simulink model "simulink_drone_offline_kalman"  (R2024b)
settings: Solver=VariableStepAuto  StartTime=0.0  StopTime=20  RelTol=1e-3
values from neighbouring files (symbols this model uses):
  A = A_numeric    [calculate_kalman_gain.m]    (also in expanded_drone_dynamics.m = [1 0 0 0 0 0 dt 0 0 0 0 0 0.5*(dt^2) 0 0 0 0 0; lqr_computation.m = jacobian(f, X); new_strategy.m = jacobian(f, X); new_strategy_integrated.m = jacobian(f, X))
  B = B_numeric    [calculate_kalman_gain.m]    (also in lqr_computation.m = jacobian(f, U); new_strategy.m = jacobian(f, U); new_strategy_integrated.m = jacobian(f, U); offline_kalman_expanded.m)
  barometer_sample_time = 1/100    (= 0.01)    [simulink_vars.m]
  barometer_variance = [0.0625]    [simulink_vars.m]
  C = C_imu    [offline_kalman_expanded.m]
  C_barometer = [0 0 1 0 0 0 0 0 0 0 0 0 0 0 0 0 0 0]    [offline_kalman_expanded.m]
  C_gps = [1 0 0 0 0 0 0 0 0 0 0 0 0 0 0 0 0 0 ... (first row only)    [offline_kalman_expanded.m]
  g = params.g    [drone_dynamics.m]    (also in expanded_drone_dynamics.m; lqr_computation.m = 9.807; new_strategy.m; new_strategy_integrated.m)
  G_hov = [ 0 0 0 0 0 0 1 0 ]    [lqr_computation.m]    (also in new_strategy.m = [1 0 0 0 0 0 0 0]; new_strategy_integrated.m = [1 0 0 0 0 0 0 0])
  G_pos = [ 1 0 0 0 ... (first row only)    [lqr_computation.m]    (also in new_strategy.m = [1 0 0 0; new_strategy_integrated.m = [1 0 0 0)
  gps_sample_time = 1/20    (= 0.05)    [simulink_vars.m]
  gps_variance = 0.0025 * ones(1,3)    [simulink_vars.m]
  imu_drift = [0.0,0.0,0.0,0.00,0.00,0.00,0.0,0.0,0.0]    [simulink_vars.m]
  imu_sample_time = 1/100    (= 0.01)    [simulink_vars.m]
  imu_variance = [0.0037,0.0037,0.0037,0.1225,0.1225,0.1225,0.0029,0.0029,0.0029]    [simulink_vars.m]
  K_att = lqr(sys_red_int, Q, R)    [new_strategy.m]    (also in new_strategy_integrated.m)
  K_hor = lqr(sys_hor_int, Q_hor, R_hor)    [new_strategy.m]    (also in new_strategy_integrated.m)
  kf = round( kf, 5 )    [offline_kalman_expanded.m]
  kf_100 = round(kf_100, 5)    [calculate_kalman_gain.m]    (also in offline_kalman_expanded.m = round( kf_100, 5 ))
  kf_20 = round(kf_20, 5)    [calculate_kalman_gain.m]    (also in offline_kalman_expanded.m = round( kf_20, 5 ))
  params = struct()    [simulink_vars.m]
  params_control = [m; Jx; Jy; Jz; c; r; g]    [new_strategy.m]    (also in new_strategy_integrated.m)
  stationary_wt = sqrt(weight/(Kt * 2))    [simulink_vars.m]
  X0 = [0;0;0; 0;0;0; 0;0;0; 0;0;0]    [new_strategy.m]    (also in new_strategy_integrated.m; simulink_vars.m = [0;0;3; 0;0;0; 0;0;0; 0;0;0])
undefined symbols (not defined in the file or in its folder): B_kinematic
settings Model: Creator=dp271  LastModifiedBy=dp271

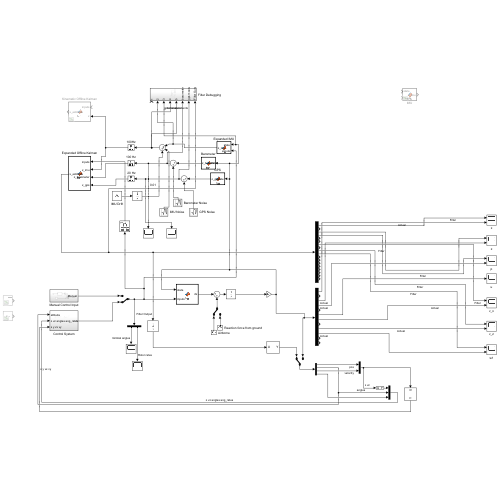
[thumbnail: Simulink's stored preview of the top-level diagram]
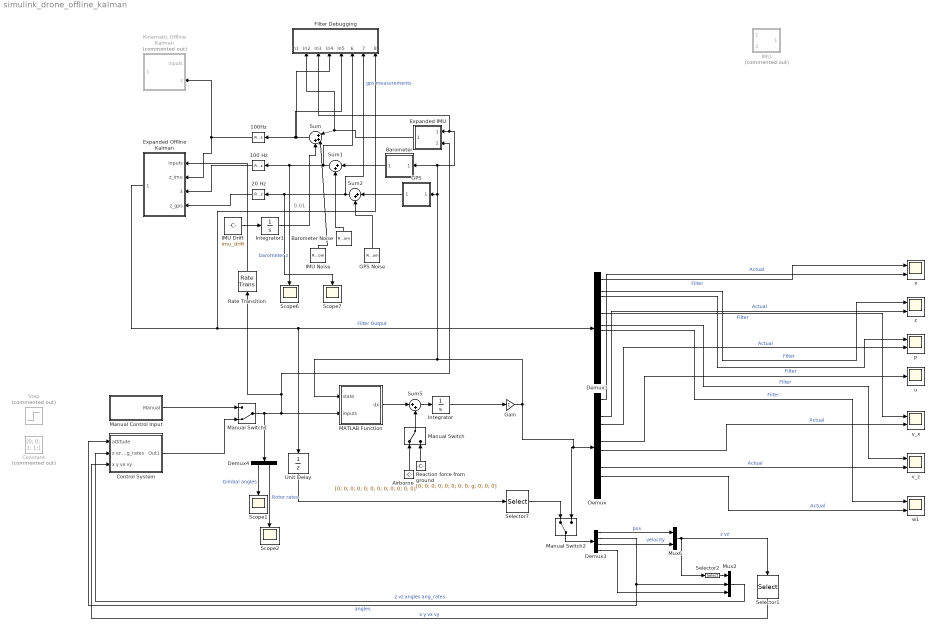
== system simulink_drone_offline_kalman ==
  note: 0.01
  " 20 Hz" : RateTransition  OutPortSampleTime=gps_sample_time
  100 Hz : RateTransition  OutPortSampleTime=barometer_sample_time
  100Hz : RateTransition  OutPortSampleTime=imu_sample_time
  Airborne : Constant  Value=[0; 0; 0; 0; 0; 0; 0; 0; 0; 0; 0; 0]
  Barometer : MATLAB Function  TreatAsAtomicUnit=on
  Barometer Noise : RandomNumber  Variance=barometer_variance  SampleTime=barometer_sample_time
  Constant : Constant  Commented=on  Value=[0; 0; 1; 1;]
  Control System : Subsystem
  Demux : Demux  Outputs=12
  Demux1 : Demux  Outputs=18
  Demux3 : Demux
  Demux4 : Demux  Outputs=2
  Expanded IMU : MATLAB Function  TreatAsAtomicUnit=on
  Expanded Offline Kalman : MATLAB Function  TreatAsAtomicUnit=on
  Filter Debugging : Subsystem
  GPS : MATLAB Function  TreatAsAtomicUnit=on
  GPS Noise : RandomNumber  Mean=zeros(3,1)  Variance=gps_variance  SampleTime=gps_sample_time
  Gain : Gain
  IMU : MATLAB Function  Commented=on  TreatAsAtomicUnit=on
  IMU Drift : Constant  Value=imu_drift  SampleTime=imu_sample_time
  IMU Noise : RandomNumber  Mean=zeros(9,1)  Variance=imu_variance  SampleTime=imu_sample_time
  Integrator : Integrator  InitialCondition=zeros(12,1)
  Integrator1 : Integrator  InitialCondition=zeros(9,1)
  Kinematic Offline Kalman : MATLAB Function  Commented=on  TreatAsAtomicUnit=on
  MATLAB Function : MATLAB Function  TreatAsAtomicUnit=on
  Manual Control Input : Subsystem
  Manual Switch : ManualSwitch
  Manual Switch1 : ManualSwitch  CurrentSetting=0
  Manual Switch2 : ManualSwitch
  Mux2 : Mux  Inputs=3
  Mux6 : Mux  Inputs=2
  Rate Transition : RateTransition  OutPortSampleTime=0.01
  Reaction force from ground : Constant  Value=[0; 0; 0; 0; 0; 0; 0; 0; g; 0; 0; 0]
  Scope{1..2,6..7} (4 alike) : Scope
  Selector1 : Selector  InputPortWidth=6  IndexOptions=Index vector (dialog)  Indices=[1 2 4 5]  OutputSizes=1
  Selector2 : Selector  InputPortWidth=6  IndexOptions=Index vector (dialog)  Indices=[3 6]  OutputSizes=1
  Selector7 : Selector  InputPortWidth=18  IndexOptions=Index vector (dialog)  Indices=[1 2 3 4 5 6 7 8 9 10 11 12]  OutputSizes=1
  Step : Step  Commented=on  Time=5  Before=stationary_wt  After=stationary_wt  SampleTime=0
  Sum : Sum  Inputs=|+++
  Sum1 : Sum  Inputs=|++
  Sum2 : Sum  Inputs=|++
  Sum5 : Sum  Inputs=|++
  Unit Delay : UnitDelay  InitialCondition=zeros(18,1)  SampleTime=0.01  HasFrameUpgradeWarning=on
  p : Scope  NumInputPorts=2
  u : Scope
  v_x : Scope  NumInputPorts=2
  v_z : Scope  NumInputPorts=2
  w1 : Scope  NumInputPorts=2
  x : Scope  NumInputPorts=2
  z : Scope  NumInputPorts=2
  wires:
  " 20 Hz"/1 -> Expanded Offline Kalman/4(z_gps)
  Demux1/1 -> x/1  "Filter"
  Demux/3 -> z/2  "Actual"
  Demux1/7 -> v_x/1  "Filter"
  Demux1/3 -> z/1  "Filter"
  IMU Drift/1 -> Integrator1/1
  Sum1/1 -> 100 Hz/1, Scope6/1, Filter Debugging/6(barometer z)  "barometer z"
  Demux/4 -> p/2  "Actual"
  Demux1/9 -> v_z/1  "Filter"
  Integrator1/1 -> Sum/3
  Barometer Noise/1 -> Sum1/2
  Demux/7 -> v_x/2  "Actual"
  Sum2/1 -> Filter Debugging/7(gps measurements), Scope7/1, " 20 Hz"/1  "gps measurements"
  GPS Noise/1 -> Sum2/2
  Demux/1 -> x/2  "Actual"
  Demux/9 -> v_z/2  "Actual"
  Sum/1 -> 100Hz/1, Filter Debugging/5(In5), Filter Debugging/4(In4)
  Demux1/4 -> p/1  "Filter"
  IMU Noise/1 -> Sum/2
  GPS/1(z_gps) -> Sum2/1
  100Hz/1 -> Expanded Offline Kalman/2(z_imu), Kinematic Offline Kalman/2(z)
  Expanded Offline Kalman/1(x_estimate) -> Demux1/1, Unit Delay/1, Filter Debugging/8(Filter Output)  "Filter Output"
  Barometer/1(z_barometer) -> Sum1/1
  100 Hz/1 -> Expanded Offline Kalman/3(z_barometer)
  Rate Transition/1 -> Expanded Offline Kalman/1(inputs)
  Gain/1 -> Demux/1, Manual Switch2/2, GPS/1(state), Filter Debugging/3(In3), Expanded IMU/1(state), Barometer/1(state), MATLAB Function/1(state)
  Demux1/10 -> w1/1  "Filter"
  Demux/10 -> w1/2  "Actual"
  MATLAB Function/1(dx) -> Sum5/1
  Sum5/1 -> Integrator/1
  Expanded IMU/1(z_imu) -> Filter Debugging/2(In2), Sum/1
  Integrator/1 -> Gain/1
  Manual Switch/1 -> Sum5/2
  Airborne/1 -> Manual Switch/1
  Reaction force from ground/1 -> Manual Switch/2
  Manual Switch1/1 -> Expanded IMU/2(inputs), Rate Transition/1, MATLAB Function/2(inputs), Demux4/1
  Demux3/2 -> Control System/1(attitude), Mux2/2  "angles"
  Demux3/4 -> Mux2/3
  Demux3/1 -> Mux6/1  "pos"
  Demux3/3 -> Mux6/2  "velocity"
  Mux6/1 -> Selector1/1, Selector2/1  "z vz"
  Selector2/1 -> Mux2/1
  Demux4/1 -> Scope1/1  "Gimbal angles"
  Demux4/2 -> Scope2/1  "Rotor rates"
  Control System/1(Out1) -> Manual Switch1/2
  Mux2/1 -> Control System/2(z vz angles ang_rates)  "z vz angles ang_rates"
  Selector1/1 -> Control System/3(x y vx vy)  "x y vx vy"
  Demux/6 -> u/1
  Manual Switch2/1 -> Demux3/1
  Unit Delay/1 -> Selector7/1
  Selector7/1 -> Manual Switch2/1
  Manual Control Input/1(Manual) -> Manual Switch1/1

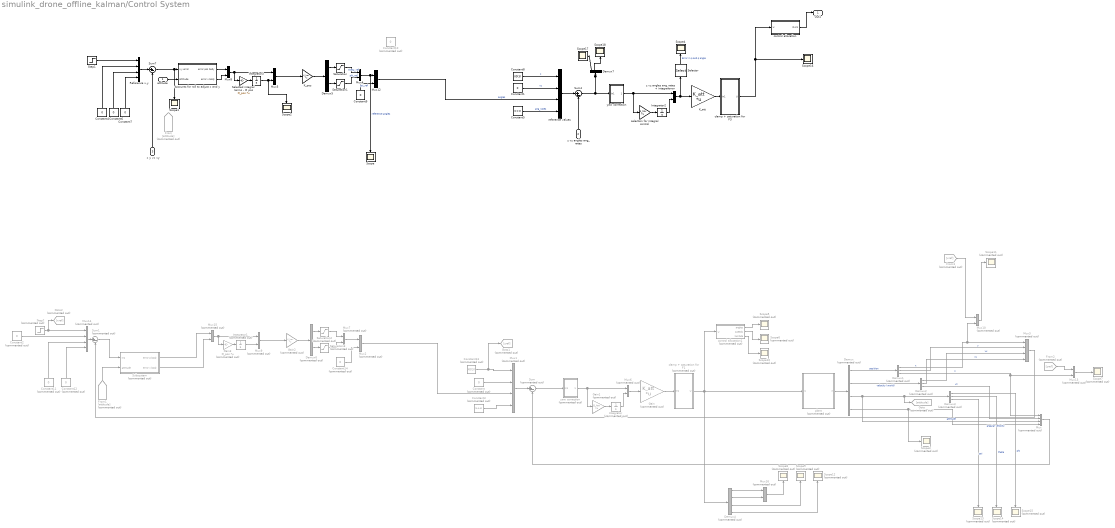
== system simulink_drone_offline_kalman/Control System ==
  attitude : Inport
  z vz angles ang_rates : Inport  Port=2
  x y vx vy : Inport  Port=3
  Accounts for roll to adjust x and y : Subsystem
  Constant{,2,10..12,14} (6 alike) : Constant  Commented=on  Value=0
  Constant{1,4,6..7,9} (5 alike) : Constant  Value=0
  Constant13 : Constant  Commented=on  Value=X0(3)
  Constant3 : Constant  Commented=on  Value=[0;0;0]  VectorParams1D=off
  Constant5 : Constant  Value=[0;0;0]  VectorParams1D=off
  Constant8 : Constant  Value=X0(3)
  Demux : Demux  Commented=on
  Demux1 : Demux  Commented=on  Outputs=3
  Demux2 : Demux  Commented=on  Outputs=3
  Demux3 : Demux  Commented=on  Outputs=3
  Demux4 : Demux  Commented=on
  Demux5 : Demux  Outputs=2
  Demux6 : Demux  Commented=on  Outputs=2
  Demux7 : Demux
  From : From  Commented=on  GotoTag=attitude
  From1 : From  Commented=on  GotoTag=attitude
  From2 : From  Commented=on  GotoTag=zref
  From3 : From  Commented=on  GotoTag=xref
  Gain : Gain  Commented=on  Gain=K_att  Multiplication=Matrix(K*u)
  Gain1 : Gain  Commented=on  Gain=G_hov  Multiplication=Matrix(K*u)
  Gain2 : Gain  Commented=on  Gain=K_hor  Multiplication=Matrix(K*u)
  Gain3 : Gain  Commented=on  Gain=G_pos  Multiplication=Matrix(K*u)
  Goto : Goto  Commented=on  GotoTag=attitude
  Goto1 : Goto  Commented=on  GotoTag=zref
  Goto2 : Goto  Commented=on  GotoTag=xref
  Integrator : Integrator  Commented=on  InitialCondition=X0(3)
  Integrator1 : Integrator  Commented=on  InitialCondition=[X0(1); X0(2)]  UpperSaturationLimit=0.4  LowerSaturationLimit=-0.4
  Integrator2 : Integrator  InitialCondition=X0(3)
  Integrator3 : Integrator  InitialCondition=[X0(1); X0(2)]  UpperSaturationLimit=0.4  LowerSaturationLimit=-0.4
  K_att : Gain  Gain=K_att  Multiplication=Matrix(K*u)
  K_pos : Gain  Gain=K_hor  Multiplication=Matrix(K*u)
  Mux{,1,3,14} (4 alike) : Mux  Commented=on
  Mux{2,6..7,9..10,13,15..16} (8 alike) : Mux  Commented=on  Inputs=2
  Mux{4..5,8,12} (4 alike) : Mux  Inputs=2
  Reference x,y : Mux
  Saturation : Saturate  UpperLimit=0.2  LowerLimit=-0.2
  Saturation1 : Saturate  UpperLimit=0.2  LowerLimit=-0.2
  Saturation2 : Saturate  Commented=on  UpperLimit=0.2  LowerLimit=-0.2
  Saturation3 : Saturate  Commented=on  UpperLimit=0.2  LowerLimit=-0.2
  Scope{,1..2,4,16..18} (7 alike) : Scope
  Scope{3,5..15} (12 alike) : Scope  Commented=on
  Selected integral terms - G_pos : Gain  Gain=G_pos  Multiplication=Matrix(K*u)
  Selector : Selector  InputPortWidth=9  IndexOptions=Index vector (dialog)  Indices=[3 4]  OutputSizes=1
  Step1 : Step  Time=11  After=0  SampleTime=0
  Step2 : Step  Commented=on  After=0.1  SampleTime=0
  Subsystem : Subsystem  Commented=on
  Sum : Sum  Commented=on  Inputs=|+-
  Sum1 : Sum  Commented=on  Inputs=|+-
  Sum4 : Sum  Inputs=|+-
  Sum7 : Sum  Inputs=|+-
  clamp + saturation for F1 : Subsystem  Commented=on
  clamp + saturation for F3 : Subsystem
  control allocation : Subsystem
  control allocation1 : Subsystem  Commented=on
  plant : Subsystem  Commented=on
  reference values : Mux
  selection for integral control : Gain  Gain=G_hov  Multiplication=Matrix(K*u)
  yaw correction : Subsystem  Commented=on
  "yaw correction " : Subsystem
  z vz angles ang_rates + integralerror : Mux  Inputs=2
  Out1 : Outport
  wires:
  Saturation1/1 -> Mux4/2  "phi_ref"
  Demux5/1 -> Saturation/1
  Constant1/1 -> reference values/2  "vz"
  Mux8/1 -> Selected integral terms - G_pos/1, Mux5/1
  Integrator2/1 -> z vz angles ang_rates + integralerror/2
  Saturation/1 -> Mux4/1  "theta_ref"
  selection for integral control/1 -> Integrator2/1
  Sum7/1 -> Scope1/1, Accounts for roll to adjust x and y/1(x,y error)
  Mux4/1 -> Scope/1, Mux12/1  "reference angles"
  K_att/1 -> clamp + saturation for F3/1(In1)
  Accounts for roll to adjust x and y/2(error v body) -> Mux8/2
  Integrator3/1 -> Scope2/1, Mux5/2
  Mux12/1 -> reference values/3  "angles"
  z vz angles ang_rates + integralerror/1 -> Selector/1, K_att/1
  Constant4/1 -> Reference x,y/2
  Constant6/1 -> Reference x,y/3
  Sum4/1 -> Demux7/1, "yaw correction "/1(In1)
  Step1/1 -> Reference x,y/1
  z vz angles ang_rates/1 -> Sum4/2
  Constant5/1 -> reference values/4  "ang_rates"
  Constant7/1 -> Reference x,y/4
  attitude/1 -> Accounts for roll to adjust x and y/2(attitude)
  "yaw correction "/1(Out1) -> selection for integral control/1, z vz angles ang_rates + integralerror/1
  clamp + saturation for F3/1(U) -> control allocation/1(U), Scope16/1
  Accounts for roll to adjust x and y/1(error pos body) -> Mux8/1
  K_pos/1 -> Demux5/1
  Mux5/1 -> K_pos/1
  Constant9/1 -> Mux12/2  "psi_ref"
  Selected integral terms - G_pos/1 -> Integrator3/1
  Reference x,y/1 -> Sum7/1
  Demux5/2 -> Saturation1/1
  Constant8/1 -> reference values/1  "z"
  reference values/1 -> Sum4/1
  x y vx vy/1 -> Sum7/2
  control allocation/1(Out1) -> Out1/1
  Selector/1 -> Scope4/1  "Error in p and q angle"
  Constant12/1 -> Mux14/4
  From1/1 -> Subsystem/2(attitude)
  Constant/1 -> Mux1/2
  yaw correction/1(Out1) -> Gain1/1, Mux6/1
  Demux3/2 -> Scope14/1  "theta"
  Mux16/1 -> Scope8/1
  Gain1/1 -> Integrator/1
  Gain2/1 -> Demux6/1
  Demux4/1 -> Mux16/1
  Subsystem/1(error p body) -> Mux15/1
  Demux3/1 -> Scope15/1  "phi"
  Mux9/1 -> Gain2/1
  Step2/1 -> Goto2/1, Mux14/1
  Constant11/1 -> Mux14/3
  control allocation1/2(speeds) -> Scope6/1
  Constant3/1 -> Mux1/4
  Integrator1/1 -> Mux9/2
  Demux2/3 -> Mux/2  "vz"
  Demux1/2 -> Mux3/2  "y"
  Constant2/1 -> Mux14/2
  Mux7/1 -> Mux2/1
  Mux10/1 -> Scope11/1
  Mux/1 -> Sum/2
  Demux4/4 -> Scope12/1
  Constant13/1 -> Goto1/1, Mux1/1
  Gain3/1 -> Integrator1/1
  Mux6/1 -> Gain/1
  control allocation1/1(angles) -> Scope5/1
  Integrator/1 -> Mux6/2
  Mux13/1 -> Scope7/1
  plant/1(X) -> Demux/1
  Sum1/1 -> Subsystem/1(In1)
  Demux2/2 -> Mux3/4  "vy"
  Demux1/3 -> Mux13/2, Mux/1  "z"
  Saturation2/1 -> Mux7/1
  Demux/4 -> Scope3/1, Mux/4  "angular velocity"
  Mux2/1 -> Mux1/3
  Demux/1 -> Demux1/1  "position"
  Gain/1 -> clamp + saturation for F1/1(In1)
  Mux14/1 -> Sum1/1
  Demux4/2 -> Mux16/2
  Demux4/3 -> Scope9/1
  control allocation1/3(lambda) -> Scope10/1
  Mux1/1 -> Sum/1
  From2/1 -> Mux13/1
  Mux3/1 -> Sum1/2
  Demux6/1 -> Saturation2/1
  Demux3/3 -> Scope13/1  "psi"
  Subsystem/2(error v body) -> Mux15/2
  Mux15/1 -> Gain3/1, Mux9/1
  From3/1 -> Mux10/1
  Saturation3/1 -> Mux7/2
  Demux/2 -> Demux2/1  "velocity (world)"
  Demux2/1 -> Mux3/3  "vx"
  Demux6/2 -> Saturation3/1
  Demux/3 -> Mux/3, Demux3/1, Goto/1  "attitude"
  Demux1/1 -> Mux10/2, Mux3/1  "x"
  Constant14/1 -> Mux2/2
  Sum/1 -> yaw correction/1(In1)
  clamp + saturation for F1/1(U) -> plant/1(U), control allocation1/1(U), Demux4/1
  Demux7/1 -> Scope17/1
  Demux7/2 -> Scope18/1

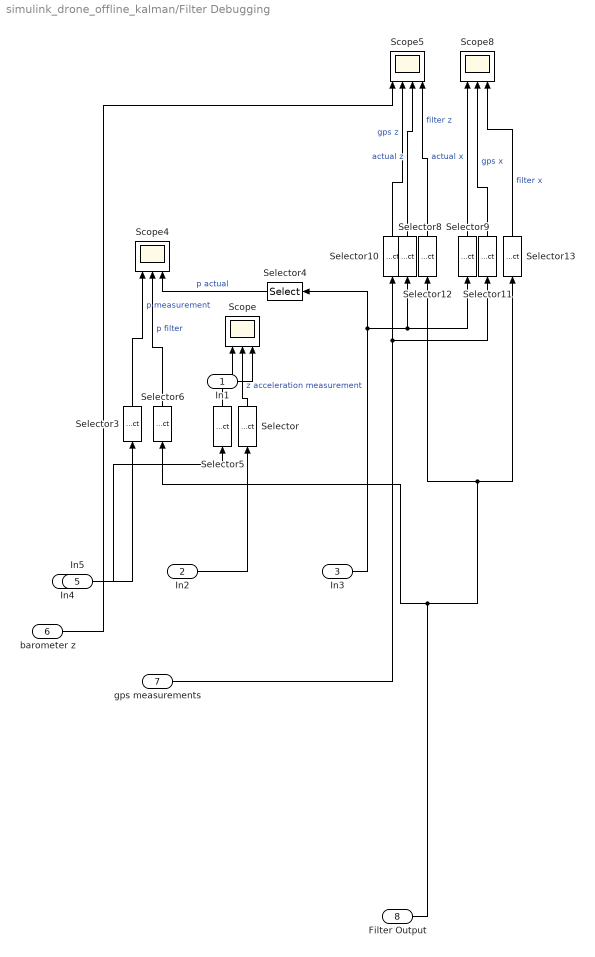
== system simulink_drone_offline_kalman/Filter Debugging ==
  In1 : Inport
  In2 : Inport  Port=2
  In3 : Inport  Port=3
  In4 : Inport  Port=4
  In5 : Inport  Port=5
  barometer z : Inport  Port=6
  gps measurements : Inport  Port=7
  Filter Output : Inport  Port=8
  Scope : Scope  NumInputPorts=3
  Scope4 : Scope  NumInputPorts=3
  Scope5 : Scope  NumInputPorts=4
  Scope8 : Scope  NumInputPorts=3
  Selector : Selector  InputPortWidth=9  IndexOptions=Index vector (dialog)  Indices=[6]  OutputSizes=1
  Selector10 : Selector  InputPortWidth=3  IndexOptions=Index vector (dialog)  Indices=[3]  OutputSizes=1
  Selector11 : Selector  InputPortWidth=3  IndexOptions=Index vector (dialog)  Indices=[1]  OutputSizes=1
  Selector12 : Selector  InputPortWidth=18  IndexOptions=Index vector (dialog)  Indices=[3]  OutputSizes=1
  Selector13 : Selector  InputPortWidth=18  IndexOptions=Index vector (dialog)  Indices=[1]  OutputSizes=1
  Selector3 : Selector  InputPortWidth=9  IndexOptions=Index vector (dialog)  Indices=[1]  OutputSizes=1
  Selector4 : Selector  InputPortWidth=12  IndexOptions=Index vector (dialog)  Indices=[4]  OutputSizes=1
  Selector5 : Selector  InputPortWidth=9  IndexOptions=Index vector (dialog)  Indices=[6]  OutputSizes=1
  Selector6 : Selector  InputPortWidth=18  IndexOptions=Index vector (dialog)  Indices=[4]  OutputSizes=1
  Selector8 : Selector  InputPortWidth=12  IndexOptions=Index vector (dialog)  Indices=[3]  OutputSizes=1
  Selector9 : Selector  InputPortWidth=12  IndexOptions=Index vector (dialog)  Indices=[1]  OutputSizes=1
  wires:
  Filter Output/1 -> Selector13/1, Selector12/1, Selector6/1
  Selector8/1 -> Scope5/3  "actual z"
  Selector5/1 -> Scope/1
  Selector/1 -> Scope/2  "z acceleration measurement"
  Selector13/1 -> Scope8/3  "filter x"
  Selector3/1 -> Scope4/1  "p measurement"
  In3/1 -> Selector9/1, Selector8/1, Selector4/1
  Selector11/1 -> Scope8/2  "gps x"
  Selector9/1 -> Scope8/1  "actual x"
  Selector10/1 -> Scope5/2  "gps z"
  Selector4/1 -> Scope4/3  "p actual"
  gps measurements/1 -> Selector11/1, Selector10/1
  Selector6/1 -> Scope4/2  "p filter"
  In2/1 -> Selector/1
  Selector12/1 -> Scope5/4  "filter z"
  In1/1 -> Scope/3
  barometer z/1 -> Scope5/1
  In4/1 -> Selector3/1
  In5/1 -> Selector5/1

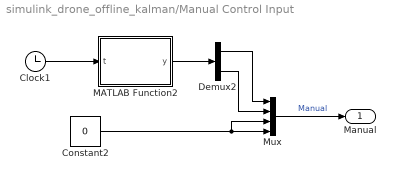
== system simulink_drone_offline_kalman/Manual Control Input ==
  Clock1 : Clock
  Constant2 : Constant  Value=0
  Demux2 : Demux  Outputs=2
  MATLAB Function2 : MATLAB Function  TreatAsAtomicUnit=on
  Mux : Mux
  Manual : Outport
  wires:
  Demux2/2 -> Mux/2
  MATLAB Function2/1(y) -> Demux2/1
  Clock1/1 -> MATLAB Function2/1(t)
  Mux/1 -> Manual/1  "Manual"
  Demux2/1 -> Mux/1
  Constant2/1 -> Mux/3, Mux/4

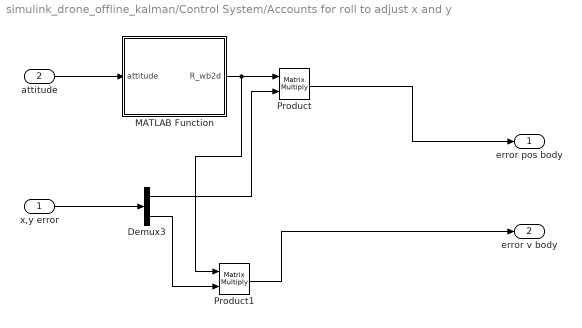
== system simulink_drone_offline_kalman/Control System/Accounts for roll to adjust x and y ==
  x,y error : Inport
  attitude : Inport  Port=2
  Demux3 : Demux  Outputs=2
  MATLAB Function : MATLAB Function  TreatAsAtomicUnit=on
  Product : Product  Multiplication=Matrix(*)
  Product1 : Product  Multiplication=Matrix(*)
  error pos body : Outport
  error v body : Outport  Port=2
  wires:
  Demux3/1 -> Product/2
  MATLAB Function/1(R_wb2d) -> Product1/1, Product/1
  x,y error/1 -> Demux3/1
  Product1/1 -> error v body/1
  Demux3/2 -> Product1/2
  Product/1 -> error pos body/1
  attitude/1 -> MATLAB Function/1(attitude)

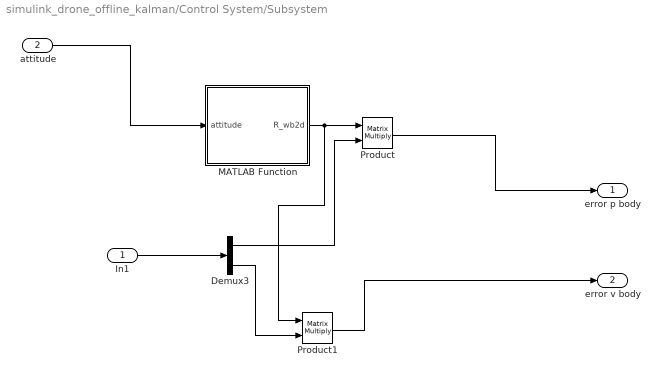
== system simulink_drone_offline_kalman/Control System/Subsystem ==
  In1 : Inport
  attitude : Inport  Port=2
  Demux3 : Demux  Outputs=2
  MATLAB Function : MATLAB Function  TreatAsAtomicUnit=on
  Product : Product  Multiplication=Matrix(*)
  Product1 : Product  Multiplication=Matrix(*)
  error p body : Outport
  error v body : Outport  Port=2
  wires:
  Demux3/1 -> Product/2
  MATLAB Function/1(R_wb2d) -> Product1/1, Product/1
  In1/1 -> Demux3/1
  Product1/1 -> error v body/1
  Demux3/2 -> Product1/2
  Product/1 -> error p body/1
  attitude/1 -> MATLAB Function/1(attitude)

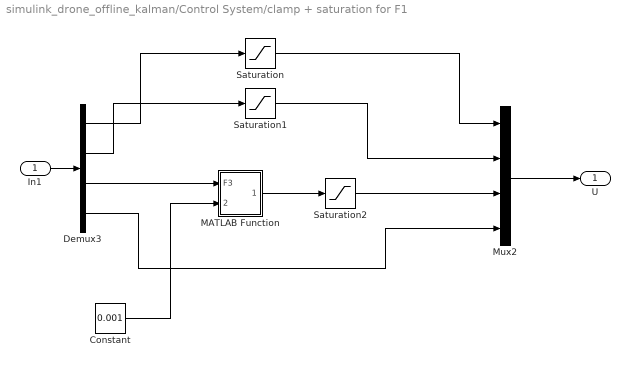
== system simulink_drone_offline_kalman/Control System/clamp + saturation for F1 ==
  In1 : Inport
  Constant : Constant  Value=0.001
  Demux3 : Demux
  MATLAB Function : MATLAB Function  TreatAsAtomicUnit=on
  Mux2 : Mux
  Saturation : Saturate  UpperLimit=3.407  LowerLimit=-3.407
  Saturation1 : Saturate  UpperLimit=3.407  LowerLimit=-3.407
  Saturation2 : Saturate  UpperLimit=19.62  LowerLimit=-19.62
  U : Outport
  wires:
  In1/1 -> Demux3/1
  Demux3/3 -> MATLAB Function/1(F3)
  Demux3/4 -> Mux2/4
  Constant/1 -> MATLAB Function/2(threshold)
  Mux2/1 -> U/1
  Demux3/1 -> Saturation/1
  Saturation/1 -> Mux2/1
  Demux3/2 -> Saturation1/1
  Saturation1/1 -> Mux2/2
  MATLAB Function/1(F3_safe) -> Saturation2/1
  Saturation2/1 -> Mux2/3

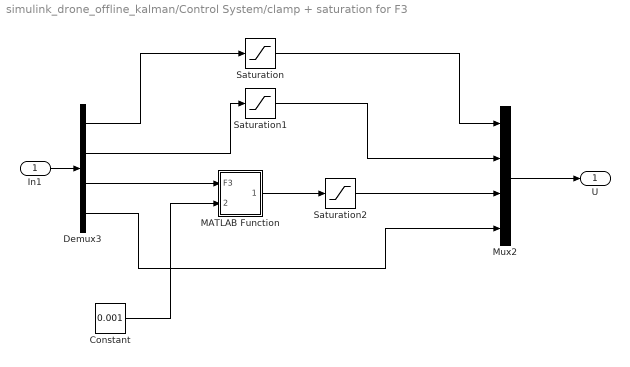
== system simulink_drone_offline_kalman/Control System/clamp + saturation for F3 ==
  In1 : Inport
  Constant : Constant  Value=0.001
  Demux3 : Demux
  MATLAB Function : MATLAB Function  TreatAsAtomicUnit=on
  Mux2 : Mux
  Saturation : Saturate  UpperLimit=3.407  LowerLimit=-3.407
  Saturation1 : Saturate  UpperLimit=3.407  LowerLimit=-3.407
  Saturation2 : Saturate  UpperLimit=19.62  LowerLimit=-19.62
  U : Outport
  wires:
  In1/1 -> Demux3/1
  Demux3/3 -> MATLAB Function/1(F3)
  Demux3/4 -> Mux2/4
  Constant/1 -> MATLAB Function/2(threshold)
  Mux2/1 -> U/1
  Demux3/1 -> Saturation/1
  Saturation/1 -> Mux2/1
  Demux3/2 -> Saturation1/1
  Saturation1/1 -> Mux2/2
  MATLAB Function/1(F3_safe) -> Saturation2/1
  Saturation2/1 -> Mux2/3

== system simulink_drone_offline_kalman/Control System/control allocation ==
  U : Inport
  MATLAB Function : MATLAB Function  TreatAsAtomicUnit=on
  Out1 : Outport
  wires:
  U/1 -> MATLAB Function/1(U)
  MATLAB Function/1(y) -> Out1/1

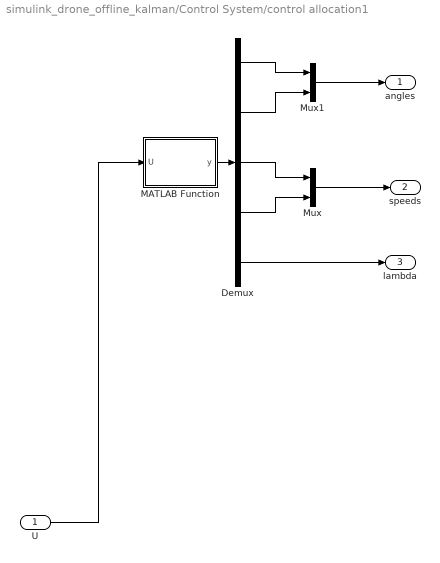
== system simulink_drone_offline_kalman/Control System/control allocation1 ==
  U : Inport
  Demux : Demux  Outputs=5
  MATLAB Function : MATLAB Function  TreatAsAtomicUnit=on
  Mux : Mux  Inputs=2
  Mux1 : Mux  Inputs=2
  angles : Outport
  speeds : Outport  Port=2
  lambda : Outport  Port=3
  wires:
  U/1 -> MATLAB Function/1(U)
  MATLAB Function/1(y) -> Demux/1
  Demux/5 -> lambda/1
  Demux/3 -> Mux/1
  Demux/4 -> Mux/2
  Mux/1 -> speeds/1
  Mux1/1 -> angles/1
  Demux/1 -> Mux1/1
  Demux/2 -> Mux1/2

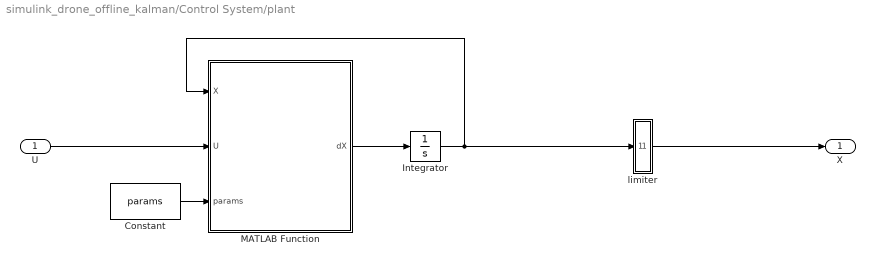
== system simulink_drone_offline_kalman/Control System/plant ==
  U : Inport
  Constant : Constant  Value=params  VectorParams1D=off
  Integrator : Integrator  InitialCondition=X0
  MATLAB Function : MATLAB Function  TreatAsAtomicUnit=on
  limiter : Subsystem
  X : Outport
  wires:
  MATLAB Function/1(dX) -> Integrator/1
  Constant/1 -> MATLAB Function/3(params)
  Integrator/1 -> limiter/1(In1), MATLAB Function/1(X)
  U/1 -> MATLAB Function/2(U)
  limiter/1(Out1) -> X/1

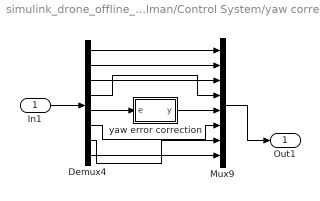
== system simulink_drone_offline_kalman/Control System/yaw correction ==
  In1 : Inport
  Demux4 : Demux  Outputs=8
  Mux9 : Mux  Inputs=8
  yaw error correction : MATLAB Function  TreatAsAtomicUnit=on
  Out1 : Outport
  wires:
  Demux4/5 -> yaw error correction/1(e)
  Demux4/4 -> Mux9/4
  Demux4/6 -> Mux9/6
  Demux4/3 -> Mux9/3
  yaw error correction/1(y) -> Mux9/5
  Demux4/8 -> Mux9/8
  Demux4/1 -> Mux9/1
  Demux4/7 -> Mux9/7
  Demux4/2 -> Mux9/2
  In1/1 -> Demux4/1
  Mux9/1 -> Out1/1

== system simulink_drone_offline_kalman/Control System/yaw correction  ==
  In1 : Inport
  Demux4 : Demux  Outputs=8
  Mux9 : Mux  Inputs=8
  yaw error correction : MATLAB Function  TreatAsAtomicUnit=on
  Out1 : Outport
  wires:
  Demux4/5 -> yaw error correction/1(e)
  Demux4/4 -> Mux9/4
  Demux4/6 -> Mux9/6
  Demux4/3 -> Mux9/3
  yaw error correction/1(y) -> Mux9/5
  Demux4/8 -> Mux9/8
  Demux4/1 -> Mux9/1
  Demux4/7 -> Mux9/7
  Demux4/2 -> Mux9/2
  In1/1 -> Demux4/1
  Mux9/1 -> Out1/1

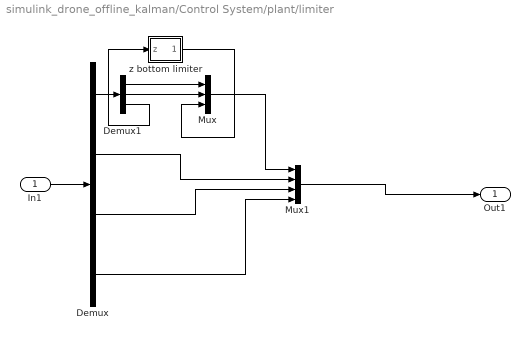
== system simulink_drone_offline_kalman/Control System/plant/limiter ==
  In1 : Inport
  Demux : Demux
  Demux1 : Demux  Outputs=3
  Mux : Mux  Inputs=3
  Mux1 : Mux
  z bottom limiter : MATLAB Function  TreatAsAtomicUnit=on
  Out1 : Outport
  wires:
  z bottom limiter/1(z_true) -> Mux/3
  Demux/2 -> Mux1/2
  Demux1/3 -> z bottom limiter/1(z)
  Demux1/1 -> Mux/1
  Mux/1 -> Mux1/1
  Demux/3 -> Mux1/3
  Demux1/2 -> Mux/2
  Demux/4 -> Mux1/4
  Demux/1 -> Demux1/1
  Mux1/1 -> Out1/1
  In1/1 -> Demux/1

== matlab function simulink_drone_offline_kalman/GPS ==
  data: state input; z_gps output
function z_gps= fcn(state)
    z_gps = gps(state);
end

== matlab function simulink_drone_offline_kalman/Control System/Accounts for roll to adjust x and y/MATLAB Function ==
  data: attitude input; R_wb2d output
function R_wb2d = fcn(attitude)

u = attitude(3);

R_wb2d = [ cos(u), sin(u);
           -sin(u), cos(u)];

end

== matlab function simulink_drone_offline_kalman/Manual Control Input/MATLAB Function2 ==
  data: t input; y output
function y = fcn(t)
    angle = 0;
    %angle = 0.1;
    y = [0;0];
    if t > 4
        y= [angle; angle]; 
    end

    % 
    % if t > 3.8 && t < 3.9
    %     y= [angle;angle];
    % elseif t > 3.9 && t < 4
    %     y= -[angle;angle];
    % else
    %     y = zeros(2,1);
    % end

== matlab function simulink_drone_offline_kalman/Control System/clamp + saturation for F3/MATLAB Function ==
  data: F3 input; F3_safe output; threshold input
function F3_safe = clamp_F3(F3, threshold)
% Prevents F3 passing through zero to avoid singularities
% threshold: the deadzone boundary (e.g. 0.001)

if F3 >= 0 && F3 < threshold
    F3_safe = threshold;
elseif F3 < 0 && F3 > -threshold
    F3_safe = -threshold;
else
    F3_safe = F3;
end

end

== matlab function simulink_drone_offline_kalman/Control System/yaw correction /yaw error correction ==
  data: e input; y output
function y = fcn(e)

    if( e > pi )
        e = e - 2* pi; 
    end

    y = e;
end

== matlab function simulink_drone_offline_kalman/Control System/control allocation/MATLAB Function ==
  data: U input; y output; params_control parameter; params parameter
function y = fcn(U, params_control, params)
F1 = U(1);
F2 = U(2);
F3 = U(3);
Mz = U(4);
Kt = params.Kt;%0.021
c = params_control(5); 

F_norm = sqrt(F1^2 + F2^2 + F3^2);

%alpha_1 = asin((F2/F_norm));
%alpha_2 = acos( F3/sqrt(F1^2 + F3^2));

alpha_1 = atan2(-F2, sqrt(F1^2 + F3^2));
alpha_2 = atan2(F1, F3);

omega_1 = sqrt( F_norm / Kt);

lambda = 1 - (Mz / (c * F3));

F_2norm = lambda * F_norm; 

omega_2 = sqrt( abs(F_2norm) / Kt);



%y = [alpha_1; alpha_2; omega_1; omega_2; lambda]; %lambda just for debugging
y = [alpha_1; alpha_2; omega_1; omega_2];
end

== matlab function simulink_drone_offline_kalman/Control System/Subsystem/MATLAB Function ==
  data: attitude input; R_wb2d output
function R_wb2d = fcn(attitude)

u = attitude(3);

R_wb2d = [ cos(u), sin(u);
           -sin(u), cos(u)];

end

== matlab function simulink_drone_offline_kalman/Control System/clamp + saturation for F1/MATLAB Function ==
  data: F3 input; F3_safe output; threshold input
function F3_safe = clamp_F3(F3, threshold)
% Prevents F3 passing through zero to avoid singularities
% threshold: the deadzone boundary (e.g. 0.001)

if F3 >= 0 && F3 < threshold
    F3_safe = threshold;
elseif F3 < 0 && F3 > -threshold
    F3_safe = -threshold;
else
    F3_safe = F3;
end

end

== matlab function simulink_drone_offline_kalman/Control System/control allocation1/MATLAB Function ==
  data: U input; y output
function y = fcn(U)
F1 = U(1);
F2 = U(2);
F3 = U(3);
Mz = U(4);
Kt = 0.021;
c = 0.05;

F_norm = sqrt(F1^2 + F2^2 + F3^2);

alpha_1 = asin((F2/F_norm));

alpha_2 = acos( F3/sqrt(F1^2 + F3^2));

omega_1 = sqrt( F_norm / Kt);

lambda = 1 - (Mz / (c * F3));

F_2norm = lambda * F_norm; 

omega_2 = sqrt( abs(F_2norm) / Kt);



y = [alpha_1; alpha_2; omega_1; omega_2; lambda];

end

== matlab function simulink_drone_offline_kalman/Control System/plant/MATLAB Function ==
  data: X input; dX output; U input; params input
function dX = rocket_eom(X, U, params)
% ROCKET_EOM  Equations of motion for VTOL rocket (Tait-Bryan ZYX)
%
% State vector X (12x1):
%   X(1)  = x       [m]       inertial position
%   X(2)  = y       [m]
%   X(3)  = z       [m]
%   X(4)  = vx      [m/s]     inertial velocity
%   X(5)  = vy      [m/s]
%   X(6)  = vz      [m/s]
%   X(7)  = phi     [rad]     roll
%   X(8)  = theta   [rad]     pitch
%   X(9)  = psi     [rad]     yaw
%   X(10) = wx      [rad/s]   body angular rates
%   X(11) = wy      [rad/s]
%   X(12) = wz      [rad/s]
%
% Input vector U (4x1):
%   U(1) = F1       [N]       thrust (main engine or gimbal)
%   U(2) = F2       [N]
%   U(3) = F3       [N]
%   U(4) = Mz       [Nm]      yaw moment

% --- Unpack states ---
% vx = X(4); vy = X(5); vz = X(6);  % not needed explicitly below
phi   = X(7);
theta = X(8);
psi   = X(9);
wx    = X(10);
wy    = X(11);
wz    = X(12);

% --- Unpack inputs ---
F1 = U(1);
F2 = U(2);
F3 = U(3);
Mz = U(4);

% --- Parameters (edit as needed) ---
m = params(1);
Jx = params(2);
Jy = params(3);
Jz = params(4);
c = params(5);
r = params(6);
g = params(7);
% --- Precompute trig ---
sphi = sin(phi);   cphi = cos(phi);
sth  = sin(theta); cth  = cos(theta); tth = tan(theta);
spsi = sin(psi);   cpsi = cos(psi);

% --- Shared factor from your symbolic output ---
k = (Mz/(F3*c) - 2);

% --- Position derivatives (= velocities) ---
dx = X(4);
dy = X(5);
dz = X(6);

% --- Velocity derivatives (forces / m) ---
dvx = -(F3*k*(sphi*spsi + cphi*cpsi*sth) ...
       - F2*k*(cphi*spsi - cpsi*sphi*sth) ...
       + F1*cpsi*cth*k) / m;

dvy = -(F2*k*(cphi*cpsi + sphi*spsi*sth) ...
       - F3*k*(cpsi*sphi - cphi*spsi*sth) ...
       + F1*cth*spsi*k) / m;

dvz = -g - (F3*cphi*cth*k ...
           - F1*sth*k ...
           + F2*cth*sphi*k) / m;

% --- Euler angle derivatives (kinematics) ---
dphi   = wx + wz*cphi*tth + wy*sphi*tth;
dtheta =      wy*cphi     - wz*sphi;
dpsi   =     (wz*cphi + wy*sphi) / cth;

% --- Angular rate derivatives (Euler's equations) ---
dwx = (F2*r + Jy*wy*wz - Jz*wy*wz) / Jx;
dwy = -(F1*r + Jx*wx*wz - Jz*wx*wz) / Jy;
dwz = (Mz + Jx*wx*wy - Jy*wx*wy) / Jz;

% --- Assemble output ---
if (X(3) > 0 || dvz > 0)
    % return all derivs
    dX = [dx; dy; dz; dvx; dvy; dvz; dphi; dtheta; dpsi; dwx; dwy; dwz];
else
    dX = [0; 0; 0; 0; 0; 0; dphi; dtheta; dpsi; dwx; dwy; dwz];
end

== matlab function simulink_drone_offline_kalman/Control System/plant/limiter/z bottom limiter ==
  data: z input; z_true output
function z_true = fcn(z)
if (z < 0)
    z_true = 0;
else
    z_true = z;
end

== matlab function simulink_drone_offline_kalman/Control System/yaw correction/yaw error correction ==
  data: e input; y output
function y = fcn(e)

    if( e > pi )
        e = e - 2* pi; 
    end

    y = e;
end

== matlab function simulink_drone_offline_kalman/Kinematic Offline Kalman ==
  data: inputs input; x_estimate output; z input; A parameter; B parameter; kf parameter; C parameter; B_kinematic parameter
function x_estimate = fcn(inputs, z, A, B, kf, C, B_kinematic)
    persistent x_internal
    
    % State vectors used for derivation
    %nw = [p q u].';     % Attitude (world frame)
    %wb = [wx wy wz].';  % Angular velocity (body frame) 
    %pw = [x y z].';     % Position (world frame)
    %vb = [vx vy vz].';  % Velocity (body frame) 
    
    %SWITCHED TO WORKING IN WORLD FRAME


    dt = 0.01;
    if isempty(x_internal)
        x_internal = zeros(12,1);
    end
    
    % prediction update
    %x_pred_dot = A * x_internal + B_numeric * inputs;

    p = x_internal(4); q = x_internal(5); u = x_internal(6);     
    % Rotation matrix from body to world frame, input: roll, pitch, yaw
    R = [cos(q)*cos(u), sin(p)*sin(q)*cos(u)-cos(p)*sin(u), cos(p)*sin(q)*cos(u)+sin(p)*sin(u) ;
         cos(q)*sin(u), sin(p)*sin(q)*sin(u)+cos(p)*cos(u), cos(p)*sin(q)*sin(u)-sin(p)*cos(u) ;
         -sin(q),       sin(p)*cos(q),                      cos(p)*cos(q)                     ];

    g = 9.807;
    acc_total_world = R*z(4:6) - [0; 0; g];
    x_pred = A * x_internal + B_kinematic * acc_total_world + B * inputs; %Kinematic model
    %x_pred = x_internal + x_pred_dot;
    
    % measurement update
    x_internal = x_pred + kf * ([z(1:3); z(7:9)] - C * x_pred); %No dt here because dlqe should account for it
    
    x_estimate = x_internal;
    %x_estimate(7:9) = R * x_internal(7:9);
end

== matlab function simulink_drone_offline_kalman/MATLAB Function ==
  data: state input; inputs input; dx output; params parameter
function dx = fcn(state, inputs, params)

    dx = drone_dynamics(state, inputs, params);

end

== matlab function simulink_drone_offline_kalman/Barometer ==
  data: state input; z_barometer output
function z_barometer= fcn(state)
    z_barometer = barometer(state);
end

== matlab function simulink_drone_offline_kalman/Expanded Offline Kalman ==
  data: inputs input; z_imu input; z_barometer input; z_gps input; x_estimate output; kf_20 parameter; kf_100 parameter; params parameter; C_barometer parameter; C_gps parameter
function x_estimate = fcn(inputs, z_imu, z_barometer, z_gps, kf_20, kf_100, params, C_barometer, C_gps)
    persistent x_internal last_gps_val

    %initialises internal state estimate + last gps value
    if isempty(x_internal)
        x_internal = zeros(18,1);
    end

    if isempty(last_gps_val)
        last_gps_val = zeros(3,1);
    end

    [x_internal, last_gps_val] = kalman_filter(x_internal, inputs, last_gps_val, z_imu, z_barometer, z_gps, kf_20, kf_100, params, C_barometer, C_gps);
    
    x_estimate = x_internal;

    
end

== matlab function simulink_drone_offline_kalman/Expanded IMU ==
  data: state input; z_imu output; inputs input; params parameter
function z_imu = fcn(state, inputs, params)
    %% Right now I can;t use expanded_imu because that function takes in 18x1 state vector    


    % Extract States 
    % Euler Angles (Roll, Pitch, Yaw)
    p = state(4); q = state(5); u = state(6); 
    % Angular Rates (p, q, r)
    wx = state(10); wy = state(11); wz = state(12);

    % Extract control inputs
    a1 = inputs(1); a2 = inputs(2); wt1 = inputs(3); wt2 = inputs(4); % angles, rotation rates

    % Drone Constants
    m  = params.m;
    g  = params.g;
    Kt = params.Kt;
                
    % Magnitude of force from rotor
    Ft = Kt * (wt1^2 + wt2 ^2);
    
    % Direction of gimbal
    X_force = [sin(a2) * cos(a1);
               -sin(a1);
               cos(a2) * cos(a1)];
    
    % Force from rotors
    fb = Ft * X_force;
        
    % State vectors used for derivation
    nw = [p q u].';     % Attitude (world frame)
    wb = [wx wy wz].';  % Angular velocity (body frame) 

    vb_dot = 1/m * ( fb);

    z_imu = [nw; % angular position
            vb_dot; % linear acceleration in body frame
            wb]; % angular velcity

end

== matlab function simulink_drone_offline_kalman/IMU ==
  data: state input; z_imu output; inputs input
function z_imu = fcn(state, inputs)
    z_imu = imu(state, inputs);
end
